simulink model "mpcSetpointCvxgen"  (Simulink 7.9)
settings: Solver=ode4  StartTime=0.0  StopTime=200  RelTol=1e-3
values from neighbouring files (symbols this model uses):
  A = params.A    [cvxsolve.m]
  B = params.B    [cvxsolve.m]
  dt = 0.5    [prepFourMasses.m]    (also in prepSixMasses.m; prepSoftKS.m)
  Ed_block = Ef_block    [prepFourMasses.m]    (also in prepSixMasses.m; prepSoftKS.m)
  Ef_block = zeros(2*n,1)    [prepFourMasses.m]    (also in prepSixMasses.m; prepSoftKS.m)
  ef_block = Ef_block    [prepFourMasses.m]    (also in prepSixMasses.m; prepSoftKS.m)
  f = params.f    [cvxsolve.m]    (also in prepFourMasses.m = [0.5*ones(4,1)]; prepSixMasses.m = [.5*ones(6,1)]; prepSoftKS.m = [0.5*ones(6,1)])
  Ff = params.Ff    [cvxsolve.m]    (also in prepFourMasses.m = [[1] zeros(1,7)]; prepSixMasses.m = [[1;1] zeros(2,11)]; prepSoftKS.m = [[1;1] zeros(2,11)])
  ff = params.ff    [cvxsolve.m]    (also in prepFourMasses.m = [xmax]; prepSixMasses.m = [.3; .3]; prepSoftKS.m = [.3; .3])
  fs = params.fs    [cvxsolve.m]    (also in prepFourMasses.m = [xmax*ones(4,1) ]*100; prepSixMasses.m = [1*ones(12,1) ]*100; prepSoftKS.m = [0.3*ones(12,1) ]*100)
  Fu = params.Fu    [cvxsolve.m]    (also in prepFourMasses.m = [eye(2); -eye(2) ]; prepSixMasses.m = [eye(3); -eye(3) ]; prepSoftKS.m = [eye(3); -eye(3) ])
  Fus = [zeros(4,2)]    [prepFourMasses.m]    (also in prepSixMasses.m = [zeros(12,3)]; prepSoftKS.m = [zeros(12,3)])
  Fx = [zeros(4,8)]    [prepFourMasses.m]    (also in prepSixMasses.m = [zeros(6,12)]; prepSoftKS.m = [zeros(6,12)])
  Fxs = params.Fxs    [cvxsolve.m]    (also in prepFourMasses.m = [eye(4) zeros(4)]*100; prepSixMasses.m = [eye(6) zeros(6); prepSoftKS.m = [eye(6) zeros(6))
  g = [r; repmat([q;r],T-1,1); qf]    [prepFourMasses.m]    (also in prepSixMasses.m; prepSoftKS.m)
  gt = kron(ones(T,1),[zeros(1,n); -2*Q])    [prepFourMasses.m]    (also in prepSixMasses.m; prepSoftKS.m)
  H = blkdiag(R,kron(eye(T-1),blkdiag(Q,R)),Qf)    [prepFourMasses.m]    (also in prepSixMasses.m; prepSoftKS.m)
  m = size(B,2)    [prepFourMasses.m]    (also in prepSixMasses.m; prepSoftKS.m)
  n = size(A,1)    [prepFourMasses.m]    (also in prepSixMasses.m; prepSoftKS.m)
  Q = params.Q    [cvxsolve.m]    (also in prepFourMasses.m = eye(8); prepSixMasses.m = eye(12); prepSoftKS.m = eye(12))
  R = params.R    [cvxsolve.m]    (also in prepFourMasses.m = eye(2); prepSixMasses.m = eye(3); prepSoftKS.m = eye(3))
  T = 11    [prepFourMasses.m]    (also in prepSixMasses.m = 31; prepSoftKS.m = 10)
undefined symbols (not defined in the file or in its folder): Qf
libraries: simulink x1
settings Model: Creator=aeagr  LastModifiedBy=aeagr
settings DebuggingCC: StrictBusMsg=Warning
settings GRTTargetCC: CombineOutputUpdateFcns=off  GRTInterface=on

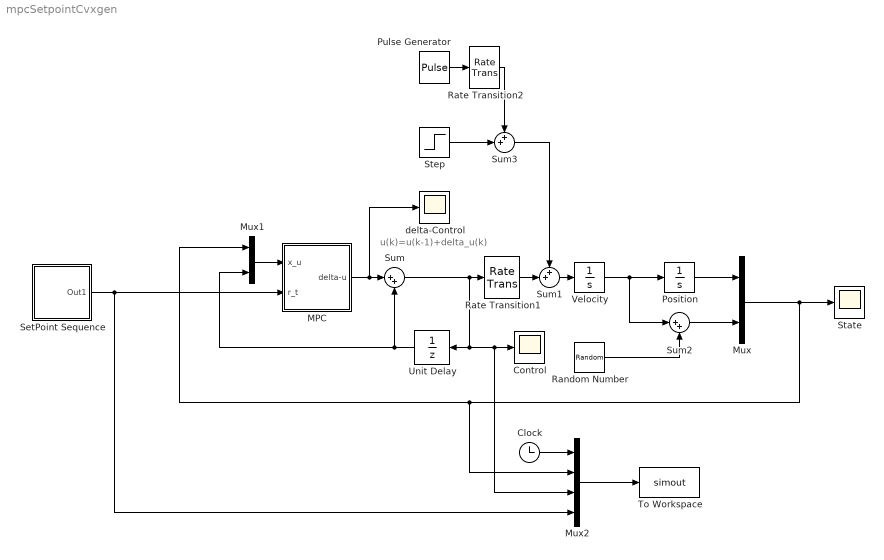
== system mpcSetpointCvxgen ==
  note: u(k)=u(k-1)+delta_u(k)
  Clock : Clock
  Control : Scope
      settings: TimeRange=240  YMin=-0.4  YMax=0.35
  MPC : Subsystem  RequirementInfo="{}  %GIDa_0c6e92d2_bf34_4970_87ae_4e32833bf9c6"  TreatAsAtomicUnit=on  SystemSampleTime=dt
      settings: RTWSystemCode=Function  RTWFcnNameOpts=Use subsystem name  RTWFileNameOpts=Use subsystem name
  Mux : Mux  Inputs=2
  Mux1 : Mux  Inputs=2
  Mux2 : Mux
  Position : Integrator
  Pulse Generator : DiscretePulseGenerator  PulseType=Time based  Amplitude=0.1  Period=200  PhaseDelay=100
  Random Number : RandomNumber  Variance=0.000000001  SampleTime=dt
  Rate Transition1 : RateTransition
  Rate Transition2 : RateTransition
  SetPoint Sequence : Subsystem
  State : Scope
      settings: TimeRange=200  YMin=-1  YMax=14
  Step : Step  Time=100  After=0.01  SampleTime=0
  Sum : Sum  Inputs=|++
  Sum1 : Sum  Inputs=++|
  Sum2 : Sum  Inputs=|++
  Sum3 : Sum  Inputs=++|
  To Workspace : ToWorkspace  VariableName=simout  SampleTime=-1
  Unit Delay : UnitDelay  SampleTime=dt
  Velocity : Integrator
  delta-Control : Scope
      settings: TimeRange=240  YMin=-0.4  YMax=0.35  SaveName=ScopeData2
  wires:
  Velocity/1 -> Position/1, Sum2/1
  Mux/1 -> State/1, Mux2/2, Mux1/1
  Position/1 -> Mux/1
  SetPoint Sequence/1(Out1) -> MPC/2(r_t), Mux2/4
  Sum/1 -> Unit Delay/1, Control/1, Mux2/3, Rate Transition1/1
  Unit Delay/1 -> Sum/2, Mux1/2
  MPC/1(delta-u) -> Sum/1, delta-Control/1
  Mux1/1 -> MPC/1(x_u)
  Sum1/1 -> Velocity/1
  Mux2/1 -> To Workspace/1
  Clock/1 -> Mux2/1
  Sum2/1 -> Mux/2
  Random Number/1 -> Sum2/2
  Rate Transition1/1 -> Sum1/2
  Step/1 -> Sum3/2
  Sum3/1 -> Sum1/1
  Pulse Generator/1 -> Rate Transition2/1
  Rate Transition2/1 -> Sum3/1

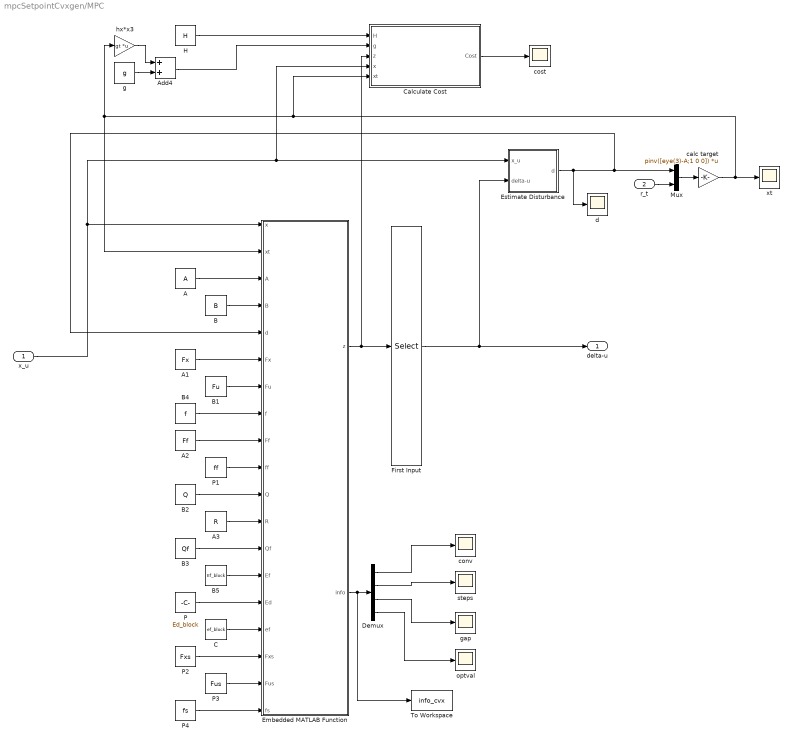
== system mpcSetpointCvxgen/MPC ==
  x_u : Inport
  r_t : Inport  Port=2
  A : Constant  Value=A
  A1 : Constant  Value=Fx
  A2 : Constant  Value=Ff
  A3 : Constant  Value=R
  Add4 : Sum
  B : Constant  Value=B
  B1 : Constant  Value=Fu
  B2 : Constant  Value=Q
  B3 : Constant  Value=Qf
  B4 : Constant  Value=f
  B5 : Constant  Value=Ef_block
  C : Constant  Value=ef_block
  Calculate Cost : Subsystem
  Demux : Demux
  Embedded MATLAB Function : MATLAB Function  TreatAsAtomicUnit=on
      settings: RTWFileNameOpts=Use subsystem name
  Estimate Disturbance : Subsystem
  First Input : Selector  InputPortWidth=T*(n+m)  IndexOptions=Index vector (dialog)  Indices=1  OutputSizes=1
  H : Constant  Value=H
  Mux : Mux  Inputs=2
  P : Constant  Value=Ed_block
  P1 : Constant  Value=ff
  P2 : Constant  Value=Fxs
  P3 : Constant  Value=Fus
  P4 : Constant  Value=fs
  To Workspace : ToWorkspace  VariableName=info_cvx  SampleTime=-1
  calc target : Gain  Gain=pinv([eye(3)-A;1 0 0])  Multiplication=Matrix(K*u)
  conv : Scope
      settings: YMin=1.65436e-24  YMax=2.75e-08  SaveName=ScopeData3
  cost : Scope
      settings: YMin=-0.25  YMax=2.5  SaveName=ScopeData8
  d : Scope
      settings: YMin=-0.00025  YMax=0.002  SaveName=ScopeData6
  g : Constant  Value=g
  gap : Scope
      settings: YMin=1.65436e-24  YMax=2.75e-08  SaveName=ScopeData5
  hx*x3 : Gain  Gain=gt  Multiplication=Matrix(K*u)
  optval : Scope
      settings: YMin=1.65436e-24  YMax=2.75e-08  SaveName=ScopeData9
  steps : Scope
      settings: YMin=1.65436e-24  YMax=2.75e-08  SaveName=ScopeData4
  xt : Scope
      settings: YMin=-0.25  YMax=2.5  SaveName=ScopeData7
  delta-u : Outport
  wires:
  First Input/1 -> delta-u/1, Estimate Disturbance/2(delta-u)
  Embedded MATLAB Function/1(z) -> First Input/1, Calculate Cost/3(z)
  H/1 -> Calculate Cost/1(H)
  x_u/1 -> Estimate Disturbance/1(x_u), Calculate Cost/4(x), Embedded MATLAB Function/1(x)
  B/1 -> Embedded MATLAB Function/4(B)
  A/1 -> Embedded MATLAB Function/3(A)
  B3/1 -> Embedded MATLAB Function/13(Qf)
  A3/1 -> Embedded MATLAB Function/12(R)
  B2/1 -> Embedded MATLAB Function/11(Q)
  A2/1 -> Embedded MATLAB Function/9(Ff)
  B1/1 -> Embedded MATLAB Function/7(Fu)
  A1/1 -> Embedded MATLAB Function/6(Fx)
  B4/1 -> Embedded MATLAB Function/8(f)
  P1/1 -> Embedded MATLAB Function/10(ff)
  Estimate Disturbance/1(d) -> Mux/1, Embedded MATLAB Function/5(d), d/1
  Mux/1 -> calc target/1
  r_t/1 -> Mux/2
  calc target/1 -> xt/1, Calculate Cost/5(xt), hx*x3/1, Embedded MATLAB Function/2(xt)
  Add4/1 -> Calculate Cost/2(g)
  B5/1 -> Embedded MATLAB Function/14(Ef)
  P2/1 -> Embedded MATLAB Function/17(Fxs)
  P3/1 -> Embedded MATLAB Function/18(Fus)
  Calculate Cost/1(Cost) -> cost/1
  g/1 -> Add4/2
  hx*x3/1 -> Add4/1
  P/1 -> Embedded MATLAB Function/15(Ed)
  C/1 -> Embedded MATLAB Function/16(ef)
  P4/1 -> Embedded MATLAB Function/19(fs)
  Embedded MATLAB Function/2(info) -> Demux/1, To Workspace/1
  Demux/1 -> conv/1
  Demux/2 -> steps/1
  Demux/3 -> gap/1
  Demux/4 -> optval/1

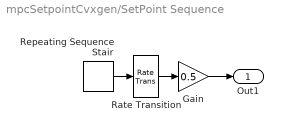
== system mpcSetpointCvxgen/SetPoint Sequence ==
  Gain : Gain  Gain=0.5
  Rate Transition : RateTransition
  Repeating Sequence Stair : simulink/Sources/Repeating Sequence Stair  OutValues=[1 0 2 0 3 0 4 0 5 0 6 0].'  tsamp=20  OutMin=[]  OutMax=[]  OutDataTypeStr=double  OutputDataTypeScalingMode=Specify via dialog  OutDataType=double  ConRadixGroup=Best Precision: Vector-wise  OutScaling=2^-12
  Out1 : Outport
  wires:
  Repeating Sequence Stair/1 -> Rate Transition/1
  Rate Transition/1 -> Gain/1
  Gain/1 -> Out1/1

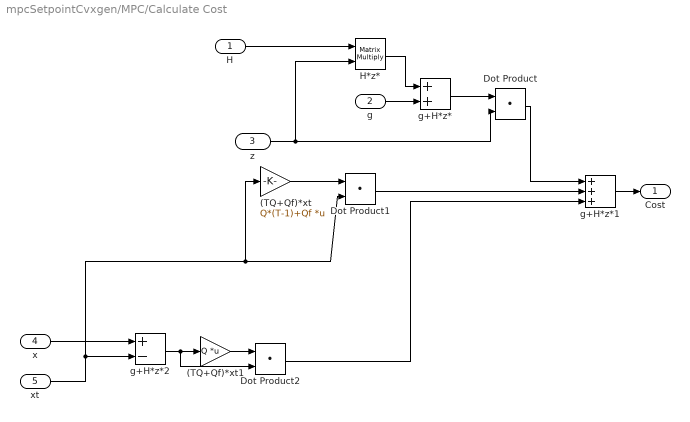
== system mpcSetpointCvxgen/MPC/Calculate Cost ==
  H : Inport
  g : Inport  Port=2
  z : Inport  Port=3
  x : Inport  Port=4
  xt : Inport  Port=5
  (TQ+Qf)*xt : Gain  Gain=Q*(T-1)+Qf  Multiplication=Matrix(K*u)
  (TQ+Qf)*xt1 : Gain  Gain=Q  Multiplication=Matrix(K*u)
  Dot Product : DotProduct  InputSameDT=on  OutDataTypeStr=Inherit: Inherit via internal rule
  Dot Product1 : DotProduct  InputSameDT=on  OutDataTypeStr=Inherit: Inherit via internal rule
  Dot Product2 : DotProduct  InputSameDT=on  OutDataTypeStr=Inherit: Inherit via internal rule
  H*z* : Product  Multiplication=Matrix(*)  RndMeth=Zero
  g+H*z* : Sum
  g+H*z*1 : Sum  Inputs=+++
  g+H*z*2 : Sum  Inputs=+-
  Cost : Outport
  wires:
  H*z*/1 -> g+H*z*/1
  g+H*z*/1 -> Dot Product/1
  (TQ+Qf)*xt/1 -> Dot Product1/1
  Dot Product/1 -> g+H*z*1/1
  Dot Product1/1 -> g+H*z*1/2
  g+H*z*2/1 -> (TQ+Qf)*xt1/1, Dot Product2/2
  (TQ+Qf)*xt1/1 -> Dot Product2/1
  Dot Product2/1 -> g+H*z*1/3
  H/1 -> H*z*/1
  g/1 -> g+H*z*/2
  z/1 -> H*z*/2, Dot Product/2
  x/1 -> g+H*z*2/1
  xt/1 -> g+H*z*2/2, (TQ+Qf)*xt/1, Dot Product1/2
  g+H*z*1/1 -> Cost/1

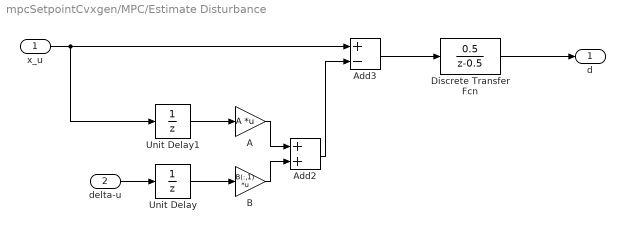
== system mpcSetpointCvxgen/MPC/Estimate Disturbance ==
  x_u : Inport
  delta-u : Inport  Port=2
  A : Gain  Gain=A  Multiplication=Matrix(K*u)
  Add2 : Sum
  Add3 : Sum  Inputs=+-
  B : Gain  Gain=B(:,1)  Multiplication=Matrix(K*u)
  Discrete Transfer Fcn : DiscreteTransferFcn  Numerator=[0.5]  Denominator=[1 -0.5]
  Unit Delay : UnitDelay  SampleTime=-1
  Unit Delay1 : UnitDelay  SampleTime=-1
  d : Outport
  wires:
  Unit Delay1/1 -> A/1
  Unit Delay/1 -> B/1
  A/1 -> Add2/1
  B/1 -> Add2/2
  Add2/1 -> Add3/2
  x_u/1 -> Unit Delay1/1, Add3/1
  delta-u/1 -> Unit Delay/1
  Add3/1 -> Discrete Transfer Fcn/1
  Discrete Transfer Fcn/1 -> d/1

== matlab function MPC/Embedded MATLAB Function ==
  data: x input double; xt input double; z output double; A input double; B input double; d input double; Fx input double; Fu input double; f input double; Ff input double; ff input double; Q input double; R input double; Qf input double; Ef input double; Ed input double; ef input double; Fxs input double; Fus input double; info output double; fs input double
function [z,info] = mpcsolve_simk(x,xt,A,B,d,Fx,Fu,f,Ff,ff,Q,R,Qf,Ef,Ed,ef,Fxs,Fus,fs)
%notcodegen
coder.extrinsic('cvxgenPointMassSolve')

z = zeros(40,1);
info = zeros(4,1);

% just call to the Matlab version
[z,info] = cvxgenPointMassSolve(x,xt,Q,R,Qf,A,B,d,Fx,Fu,f,Fxs,Fus,fs,Ef,Ed,ef,Ff,ff);
